simulink model "Chapter_4_Section_3_Model"  (R2017a)
settings: Solver=ode4  StartTime=0.0  StopTime=200  FixedStep=stp_sz  MaxStep=.0001  MinStep=.00005  RelTol=1e-7  AbsTol=1e-7  EnableMultiTasking=on
InitFcn:
  | load Chapter_4_Section_3
  | warning off
StopFcn:
  | save data.mat u_simulation v_simulation psi_simulation r_simulation npr_user_provided npr_achievable alpha_user_provided alpha_achievable stp_sz
  | clear all
  | load('data.mat')
  | delete('data.mat')
values from neighbouring files (symbols this model uses):
  A_disk = 13.2025431267    [Chapter_4_Section_3.mat]
  a_r11 = [-0.000865667853776 -0.901318756108 0.00874486630837 -0.00765974060328 0.00955717632387 0.00641813989061 -0.011076069832 0.00201248118094 -0.00501952733262 0.00315605586996 -0.00210851076531 0.0148609220099 ... (324 elements, 18x18)]    [Chapter_4_Section_3.mat]
  a_r13 = [-0.0294995912119 -4.91037219533 -0.00332739568397 0.0888755061346 -0.00681796875441 0.183812407485 0.0112008036726 0.10429312155 -0.0251601482875 -0.228675692165 0.00453476042855 0.0594697753606 ... (169 elements, 13x13)]    [Chapter_4_Section_3.mat]
  a_r15 = [-0.00127786555898 0.776225741104 -0.00474776997752 -0.00131066749835 0.0137520402687 -0.00211384579247 8.8019955143e-05 -0.00028996241197 -0.00129826872567 -0.0202543144732 0.0030370404199 -0.00453425604591 ... (169 elements, 13x13)]    [Chapter_4_Section_3.mat]
  a_r22 = [-0.000797108949019 -1.01015556887 0.00406573750109 -0.00111578544774 0.00423859757219 -0.00799128279013 0.00569024815652 -0.0167562674532 0.00334935655618 -0.000712432292804 0.00154242142086 0.00240437743229 ... (169 elements, 13x13)]    [Chapter_4_Section_3.mat]
  a_r24 = [-0.000686927823555 -0.95665602689 0.00244839898375 0.00145613314595 -0.00607023426216 0.0163996841317 0.00152022458075 -0.000736874734971 -0.00294919321651 -0.000761800577268 -0.00251686123035 -0.00197732815976 ... (169 elements, 13x13)]    [Chapter_4_Section_3.mat]
  a_r26 = [-0.194397873228 1.89810259721 -0.0873186628061 -0.241231729519 0.281206161775 -0.16994038615 -0.116565511469 -0.0496572593209 0.0216084469732 0.0912933167406 0.0299797727001 0.0314987707028 ... (169 elements, 13x13)]    [Chapter_4_Section_3.mat]
  a_r31 = [-0.00489112559449 -3.89960530455 -0.0361162658575 0.0265931197764 0.0034376033088 0.000316401308368 -0.0243996243526 0.0792200139858 -0.023187698537 -0.0726743997029 0.00400632061963 -0.0350516560041 ... (169 elements, 13x13)]    [Chapter_4_Section_3.mat]
  a_r33 = [-0.601431448276 0.50360246711 0.500115950342 -0.0452293844892 -0.0181314142185 -0.0323524621531 0.0355826051968 0.0329239610677 0.0940919952313 0.0566642992805 -0.0379178935102 0.0254835488846 ... (169 elements, 13x13)]    [Chapter_4_Section_3.mat]
  a_r35 = [-0.861988746714 -0.582511154549 0.34264856173 -0.0655310417272 -0.417167685168 0.183176698588 -0.473887691644 -0.225677727522 -0.133571139717 -0.218168843707 0.0850592077583 -0.0257492082836 ... (169 elements, 13x13)]    [Chapter_4_Section_3.mat]
  a_r42 = [-0.000411079312172 -0.966350953459 0.00419936729713 0.00358740198521 -0.00356571428733 -0.00958951498266 -0.00230062261745 -3.48708248632e-05 -0.00350313209064 -0.00772126326768 -0.0011918234528 -0.00149424537901 ... (169 elements, 13x13)]    [Chapter_4_Section_3.mat]
  a_r44 = [-0.000156115728087 -0.944139704333 -0.00242185567679 0.00620214191605 0.00232565005277 -0.00625050722164 0.00126021167241 -0.000681873506535 0.0011931592381 -0.00289361611357 -0.00138182415247 -0.00252837386868 ... (169 elements, 13x13)]    [Chapter_4_Section_3.mat]
  a_r46 = [-0.000218462457517 1.89677852742 0.00896242354968 -0.00290259500747 0.00225128874867 0.00254539590487 0.00120681433209 0.00261900930035 0.00149629742842 0.000796832004109 0.00199591847947 0.00352664402036 ... (169 elements, 13x13)]    [Chapter_4_Section_3.mat]
  a_r51 = [-0.0010898880101 0.776080724329 0.000225388678941 0.00375234840616 -0.00838297691459 -0.00447310416982 -0.0119510882322 -0.00692765468718 0.00227273345413 -0.0063592610709 0.000914007544175 0.00943534814934 ... (169 elements, 13x13)]    [Chapter_4_Section_3.mat]
  a_r53 = [-0.83377539904 0.569677058563 0.434285019976 0.157205409215 -0.397195569542 -0.255164078245 -0.141246880777 0.177451291189 -0.182828550566 0.0648162508754 0.244251292681 0.160100487197 ... (169 elements, 13x13)]    [Chapter_4_Section_3.mat]
  a_r55 = [-0.000352406331634 0.764343029796 0.00339830320259 -0.000678251137483 -0.00243783779313 -0.00215979913278 0.00196909451093 -0.00577428819561 -0.00349811892924 -0.00488920883323 0.00112064970343 0.000774855197444 ... (169 elements, 13x13)]    [Chapter_4_Section_3.mat]
  a_r62 = [-0.546519039316 -1.22303009993 0.393735845548 -0.120016588191 0.38151861373 -0.213578592342 -0.602267954372 -0.105716444149 -0.153151371839 -0.163939447448 -0.555540353196 0.0685401630267 ... (169 elements, 13x13)]    [Chapter_4_Section_3.mat]
  a_r64 = [-0.0406191100017 -5.18251105957 -0.115497941507 -0.0935821370219 0.180972853448 -0.0201998949456 -0.0698170640352 -0.0736823539521 -0.034828919888 0.0876659960431 -0.0419335596239 -0.0240984963396 ... (169 elements, 13x13)]    [Chapter_4_Section_3.mat]
  a_r66 = [-0.00276803466684 1.11530008029 0.0229779449181 0.0262185319857 0.00628472844795 0.000156167369042 -0.00250093023805 -0.0114435042874 -0.00826774415326 -0.00991601759993 -0.00812142854996 0.0148245002111 ... (169 elements, 13x13)]    [Chapter_4_Section_3.mat]
  A_rudder = 6    [Chapter_4_Section_3.mat]
  alpha_max = 0.392699081699    [Chapter_4_Section_3.mat]
  b_r11 = [-1.91804272115 -67.7547902158 12.3212653748 -6.25011871643 13.082442224 5.48501776184 -10.1596546398 2.56004852009 -4.74360113798 3.95981895348 -2.02856412397 18.3264246889 ... (18 elements, 18x1)]    [Chapter_4_Section_3.mat]
  b_r13 = [9.68113335046 8.54720242819 0.883931047444 -5.56576078332 1.72641800243 -13.8756826027 -2.702777864 -9.4621991361 5.92943514782 22.6516835054 -1.0074598861 -6.31102592982 ... (13 elements, 13x1)]    [Chapter_4_Section_3.mat]
  b_r22 = [-8.230214728 -263.156134326 24.2327808151 -4.87921448873 19.1715641288 -45.8768653263 26.6325387064 -91.9399975548 16.6663243552 -3.80929112747 7.68030110892 12.8381492859 ... (13 elements, 13x1)]    [Chapter_4_Section_3.mat]
  b_r24 = [20.6689502907 674.321335078 -41.3637763247 -19.2444203625 82.0775505272 -259.897803047 -22.2545830602 11.3827604156 43.2189922355 11.7516897475 36.9394390446 30.4503929007 ... (13 elements, 13x1)]    [Chapter_4_Section_3.mat]
  b_r26 = [206.794755218 -62.242559329 24.5666904254 184.158146246 -103.419961827 115.160111337 76.4499795128 20.3457431208 -13.1704465249 -41.5730935141 -18.1334448714 -14.4641153742 ... (13 elements, 13x1)]    [Chapter_4_Section_3.mat]
  b_r31 = [3.76230189948 5.16928151238 2.64945725635 -18.4251953385 -2.0625905672 -0.18887543415 4.20433084471 -14.07893046 13.0563354882 16.4007691754 -2.13849071942 8.28528512456 ... (13 elements, 13x1)]    [Chapter_4_Section_3.mat]
  b_r33 = [-425.265727934 16.4952177922 163.76327445 -15.539902078 -6.59006558263 -11.1862310226 12.8543123126 11.4260264426 33.8206936715 19.7626944669 -13.5783728882 8.91023495161 ... (13 elements, 13x1)]    [Chapter_4_Section_3.mat]
  b_r35 = [955.467057384 23.8174564739 -126.402446683 48.3788727465 168.435579445 -128.161344325 216.24493699 142.979450788 65.1193355403 134.911935543 -50.7648858119 13.1799100865 ... (13 elements, 13x1)]    [Chapter_4_Section_3.mat]
  b_r42 = [15.9360311823 665.959154186 -98.5777560157 -55.5400651809 61.9220987195 200.312325561 47.5124103398 0.631683490985 64.1219861023 155.750535985 22.3985447876 29.803792586 ... (13 elements, 13x1)]    [Chapter_4_Section_3.mat]
  b_r44 = [-27.1891200017 -1761.50772747 -283.391471232 367.311489951 182.522124626 -579.755911925 104.353356772 -62.2376848714 99.3185259533 -260.784153955 -116.536414334 -226.454300618 ... (13 elements, 13x1)]    [Chapter_4_Section_3.mat]
  b_r46 = [-26.6906838426 431.487773123 657.709356633 -144.976364483 114.646575538 180.775978583 85.0953284375 135.592940904 78.9082960716 55.2973047721 106.740201988 241.432567993 ... (13 elements, 13x1)]    [Chapter_4_Section_3.mat]
  b_r51 = [-27.9768378982 741.05041888 2.33758926296 57.3995096963 -127.005620965 -47.2947833409 -133.876425682 -98.5907202753 26.0445243962 -88.3721242204 10.7680008324 130.122749963 ... (13 elements, 13x1)]    [Chapter_4_Section_3.mat]
  b_r53 = [949.455593416 -23.2452293814 -157.318364745 -121.412853107 173.067821874 177.10214052 64.7164189373 -120.452255472 86.0623964314 -43.0643550932 -116.39314584 -105.497696438 ... (13 elements, 13x1)]    [Chapter_4_Section_3.mat]
  b_r55 = [-217.127382907 9506.32343029 1148.82922273 -188.742556573 -694.43970838 -709.996440288 566.872400877 -1877.38940059 -1026.37679575 -1566.80129668 332.089563592 247.692614281 ... (13 elements, 13x1)]    [Chapter_4_Section_3.mat]
  b_r62 = [259.61149635 16.5485296799 -38.0095496792 45.1883806678 -40.3107166739 78.3455844965 73.5107367495 37.0054960802 51.6709447748 22.7410486275 84.4875008959 -21.9559289205 ... (13 elements, 13x1)]    [Chapter_4_Section_3.mat]
  b_r64 = [156.539833252 187.686482031 376.820920142 59.4312894666 -548.902692032 17.0176436095 70.7484878223 206.821047291 37.1716677759 -243.032149857 114.824775027 27.0037475025 ... (13 elements, 13x1)]    [Chapter_4_Section_3.mat]
  b_r66 = [-314.266256408 5285.46587095 1093.01941502 1627.30071258 387.633965073 8.0986510694 -130.443621448 -701.343286032 -436.49966457 -600.0481003 -433.735518303 884.367320612 ... (13 elements, 13x1)]    [Chapter_4_Section_3.mat]
  bettas_CQ = [0 5.39 17.77 34.97 50.79 58.7 64.55 68.33 73.49 85.2 93.11 102.75 ... (40 elements, 1x40)]    [Chapter_4_Section_3.mat]    (also in looking_up_n.m = [0 5.39 17.77 34.97 50.79 58.7 64.55 68.33 73.49 85.2 93.11 )
  bettas_CT = [0 5.37 16.73 33.6 44.63 60.82 73.22 80.46 86.3 92.15 100.41 110.74 ... (52 elements, 1x52)]    [Chapter_4_Section_3.mat]    (also in looking_up_n.m = [0 5.37 16.73 33.6 44.63 60.82 73.22 80.46 86.3 92.15 100.41)
  c_r11 = [1.91804272142 -67.7547902158 -12.3212653748 -6.25011871643 -13.082442224 5.48501776185 -10.1596546398 -2.56004852009 -4.74360113798 -3.95981895348 -2.02856412396 -18.3264246889 ... (18 elements, 1x18)]    [Chapter_4_Section_3.mat]
  c_r13 = [9.68113335045 -8.54720242824 0.883931047418 5.56576078332 1.72641800244 13.8756826027 -2.702777864 9.4621991361 5.92943514781 -22.6516835054 -1.0074598861 6.31102592982 ... (13 elements, 1x13)]    [Chapter_4_Section_3.mat]
  c_r22 = [8.23021472807 -263.156134326 -24.2327808151 -4.87921448871 19.1715641288 45.8768653263 26.6325387064 91.9399975548 16.6663243552 3.80929112749 7.68030110892 -12.8381492859 ... (13 elements, 1x13)]    [Chapter_4_Section_3.mat]
  c_r24 = [20.6689502903 -674.321335078 -41.3637763247 19.2444203625 -82.0775505271 -259.897803047 22.2545830602 11.3827604156 -43.2189922355 11.7516897475 -36.9394390446 30.4503929007 ... (13 elements, 1x13)]    [Chapter_4_Section_3.mat]
  c_r26 = [-206.794755218 -62.2425593289 24.5666904254 -184.158146246 -103.419961827 -115.160111337 -76.4499795128 20.3457431209 13.1704465249 -41.5730935141 18.1334448714 -14.4641153742 ... (13 elements, 1x13)]    [Chapter_4_Section_3.mat]
  c_r31 = [3.76230189951 -5.16928151238 -2.64945725636 -18.4251953385 -2.0625905672 -0.188875434257 -4.2043308447 14.07893046 13.0563354882 -16.4007691754 -2.13849071943 -8.28528512456 ... (13 elements, 1x13)]    [Chapter_4_Section_3.mat]
  c_r33 = [-425.265727934 -16.4952177923 -163.76327445 15.539902078 -6.5900655826 11.1862310226 12.8543123126 -11.4260264426 33.8206936715 -19.7626944669 -13.5783728882 -8.91023495161 ... (13 elements, 1x13)]    [Chapter_4_Section_3.mat]
  c_r35 = [-955.467057384 23.8174564746 -126.402446683 -48.3788727464 168.435579445 128.161344325 216.24493699 -142.979450788 65.1193355403 -134.911935543 50.7648858119 13.1799100865 ... (13 elements, 1x13)]    [Chapter_4_Section_3.mat]
  c_r42 = [15.9360311824 -665.959154186 -98.5777560157 55.5400651809 -61.9220987195 200.312325561 47.5124103398 -0.631683490192 -64.1219861023 155.750535985 -22.3985447876 29.803792586 ... (13 elements, 1x13)]    [Chapter_4_Section_3.mat]
  c_r44 = [27.189120009 -1761.50772747 283.391471232 367.311489951 182.522124626 579.755911925 104.353356772 62.2376848713 99.3185259533 260.784153955 -116.536414334 226.454300618 ... (13 elements, 1x13)]    [Chapter_4_Section_3.mat]
  c_r46 = [26.6906838375 431.487773123 -657.709356633 -144.976364484 114.646575538 -180.775978583 -85.0953284373 135.592940904 78.9082960717 -55.297304772 106.740201988 -241.432567993 ... (13 elements, 1x13)]    [Chapter_4_Section_3.mat]
  c_r51 = [27.9768378982 741.05041888 2.33758926325 -57.3995096963 127.005620965 -47.2947833409 -133.876425682 98.5907202753 26.0445243962 88.3721242204 10.7680008324 -130.122749963 ... (13 elements, 1x13)]    [Chapter_4_Section_3.mat]
  c_r53 = [-949.455593416 -23.2452293814 -157.318364745 121.412853107 173.067821874 -177.10214052 64.7164189374 120.452255472 86.0623964314 43.0643550932 -116.39314584 105.497696438 ... (13 elements, 1x13)]    [Chapter_4_Section_3.mat]
  c_r55 = [217.12738291 9506.32343029 -1148.82922273 -188.742556576 -694.43970838 709.996440288 566.872400876 1877.38940059 -1026.37679575 1566.80129668 332.089563594 -247.69261428 ... (13 elements, 1x13)]    [Chapter_4_Section_3.mat]
  c_r62 = [-259.61149635 16.5485296799 -38.0095496792 -45.1883806678 -40.3107166739 -78.3455844965 73.5107367495 -37.0054960802 -51.6709447748 22.7410486275 84.4875008959 21.9559289205 ... (13 elements, 1x13)]    [Chapter_4_Section_3.mat]
  c_r64 = [-156.539833251 187.686482031 -376.820920142 59.4312894666 548.902692032 17.0176436097 70.7484878223 -206.82104729 37.1716677758 243.032149857 -114.824775027 27.0037475025 ... (13 elements, 1x13)]    [Chapter_4_Section_3.mat]
  c_r66 = [314.266256408 5285.46587095 1093.01941502 -1627.30071258 -387.633965073 8.09865107118 -130.443621448 701.343286032 -436.49966457 600.0481003 -433.735518303 -884.367320612 ... (13 elements, 1x13)]    [Chapter_4_Section_3.mat]
  CQs = [0.008 0.007 -0.002 -0.018 -0.037 -0.049 -0.06 -0.065 -0.068 -0.059 -0.057 -0.059 ... (40 elements, 1x40)]    [Chapter_4_Section_3.mat]    (also in looking_up_n.m = -0.1.*[-0.08 -0.07 0.02 0.18 0.37 0.49 0.6 0.65 0.68 0.59 0.)
  CTs = [0.32 0.29 0.19 0.01 -0.16 -0.46 -0.7 -0.77 -0.7 -0.63 -0.63 -0.69 ... (52 elements, 1x52)]    [Chapter_4_Section_3.mat]    (also in looking_up_n.m = [0.32 0.29 0.19 0.01 -0.16 -0.46 -0.7 -0.77 -0.7 -0.63 -0.63)
  d_r11 = 95.5285227708    [Chapter_4_Section_3.mat]
  d_r13 = -14.1628545989    [Chapter_4_Section_3.mat]
  d_r22 = 1468.51041279    [Chapter_4_Section_3.mat]
  d_r24 = -9785.77027698    [Chapter_4_Section_3.mat]
  d_r26 = -1700.92421833    [Chapter_4_Section_3.mat]
  d_r31 = -0.95522945761    [Chapter_4_Section_3.mat]
  d_r33 = 3827.81220596    [Chapter_4_Section_3.mat]
  d_r35 = -19539.5268707    [Chapter_4_Section_3.mat]
  d_r42 = -9418.04264727    [Chapter_4_Section_3.mat]
  d_r44 = 68252.1479072    [Chapter_4_Section_3.mat]
  d_r46 = -10162.1377852    [Chapter_4_Section_3.mat]
  d_r51 = 12054.4514237    [Chapter_4_Section_3.mat]
  d_r53 = -19539.5038011    [Chapter_4_Section_3.mat]
  d_r55 = 1991036.95813    [Chapter_4_Section_3.mat]
  d_r62 = -1405.47636444    [Chapter_4_Section_3.mat]
  d_r64 = -12342.2523681    [Chapter_4_Section_3.mat]
  d_r66 = 610786.440495    [Chapter_4_Section_3.mat]
  DEN = 5.34671106464e+28    [Chapter_4_Section_3.mat]
  dist_LOS = [-50 -49 -48 -47 -46 -45 -44 -43 -42 -41 -40 -39 ... (1051 elements, 1x1051)]    [Chapter_4_Section_3.mat]
  Dpr = 4.1    [Chapter_4_Section_3.mat]    (also in looking_up_n.m = u(4))
  Dw = 0.110526315789    [Chapter_4_Section_3.mat]
  dx = 10    [Chapter_4_Section_3.mat]
  dxr = 48.75    [Chapter_4_Section_3.mat]
  dy = 2    [Chapter_4_Section_3.mat]
  dz = 0.8    [Chapter_4_Section_3.mat]
  dzr = 0.514285714286    [Chapter_4_Section_3.mat]
  g = 10    [Chapter_4_Section_3.mat]
  gravity = 10    [Chapter_4_Section_3.mat]
  INDEX = [1 2 3 4 5 6 7 8 9]    [Chapter_4_Section_3.mat]
  Ix = 724554000    [Chapter_4_Section_3.mat]
  Iy = 4528460000    [Chapter_4_Section_3.mat]
  Iz = 4528460000    [Chapter_4_Section_3.mat]
  k_wave = [0.0157865285852 0.0224311321394 0.0345394916241 0.0578593033576 0.0778685019714 0.0983501894009 0.10403521245 0.134043066308 0.155236404606 0.203205074918 0.220032771713 0.262178651673 ... (20 elements, 1x20)]    [Chapter_4_Section_3.mat]
  Last_Pt_Accuracy = 30    [Chapter_4_Section_3.mat]
  LBP = 100    [Chapter_4_Section_3.mat]
  m = 7264000    [Chapter_4_Section_3.mat]
  phase = [4.61787442739 6.09845039199 5.44708367148 0.54182753101 2.30238916367 2.31974450279 4.30416083443 3.75697809799 4.95971993271 2.31003141527 1.29451121971 0.54454197722 ... (20 elements, 1x20)]    [Chapter_4_Section_3.mat]
  phi_0 = 0    [Chapter_4_Section_3.mat]
  psi_0 = 0    [Chapter_4_Section_3.mat]
  R_convrg = 220    [Chapter_4_Section_3.mat]
  radius_LOS = [166.575605377 166.637026665 166.698699321 166.760625342 166.82280675 166.885245588 166.947943925 167.010903854 167.074127493 167.137616985 167.201374499 167.265402228 ... (1051 elements, 1x1051)]    [Chapter_4_Section_3.mat]
  raw = 1000    [Chapter_4_Section_3.mat]    (also in looking_up_n.m = u(3))
  s = 0.15    [Chapter_4_Section_3.mat]
  S11 = 5.22457985714e+28    [Chapter_4_Section_3.mat]
  S13 = 3.79917831589e+26    [Chapter_4_Section_3.mat]
  S15 = -4.97006200608e+19    [Chapter_4_Section_3.mat]
  S22 = 4.58630932583e+28    [Chapter_4_Section_3.mat]
  S24 = 9.38800137353e+19    [Chapter_4_Section_3.mat]
  S26 = 1.30387886946e+18    [Chapter_4_Section_3.mat]
  S31 = 3.83422033136e+26    [Chapter_4_Section_3.mat]
  S33 = 1.77296018417e+28    [Chapter_4_Section_3.mat]
  S35 = 2.44593333777e+19    [Chapter_4_Section_3.mat]
  S42 = 8.93369784557e+19    [Chapter_4_Section_3.mat]
  S44 = 7.37931315974e+19    [Chapter_4_Section_3.mat]
  S46 = 27990784014.6    [Chapter_4_Section_3.mat]
  S51 = -4.98658939538e+19    [Chapter_4_Section_3.mat]
  S53 = 2.45188465874e+19    [Chapter_4_Section_3.mat]
  S55 = 1.18069051188e+19    [Chapter_4_Section_3.mat]
  S62 = 1.30580221388e+18    [Chapter_4_Section_3.mat]
  S64 = 23535167243.9    [Chapter_4_Section_3.mat]
  S66 = 1.18069078235e+19    [Chapter_4_Section_3.mat]
  ... (+18 more)
undefined symbols (not defined in the file or in its folder): magnitude
libraries: simulink x9
(part 3 of 6)

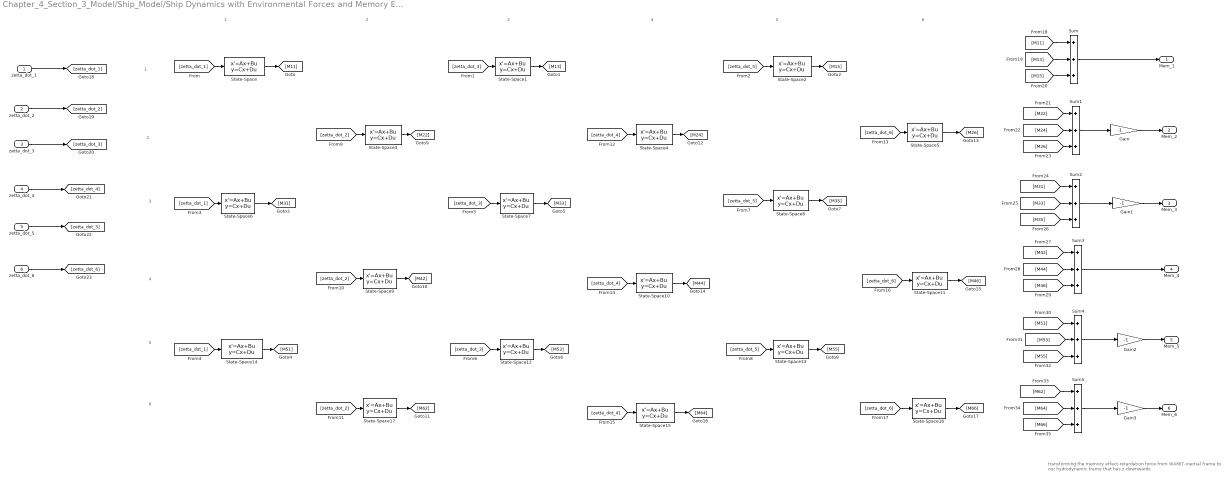
== system Chapter_4_Section_3_Model/Ship_Model/Ship Dynamics with Environmental Forces and Memory Effect/Memory effect using reduced order (13) state space representation(Kristiansen 2005)/Memory effect using reduced order (13) state space representation1 ==
  note: 1
  note: 2
  note: 3
  note: 4
  note: 5
  note: 6
  note: 1
  note: 2
  note: 3
  note: 4
  note: 5
  note: 6
  note: transforming the memory effect-retardation force from
      |  WAMIT-inertial frame to  our hydrodynamic
      |  frame that has z-downwards
  zetta_dot_1 : Inport
  zetta_dot_2 : Inport  Port=2
  zetta_dot_3 : Inport  Port=3
  zetta_dot_4 : Inport  Port=4
  zetta_dot_5 : Inport  Port=5
  zetta_dot_6 : Inport  Port=6
  Gain{,1..3} (4 alike) : Gain  Gain=-1
  State-Space : StateSpace  A=a_r11  B=b_r11  C=c_r11  D=d_r11  X0=0
  State-Space1 : StateSpace  A=a_r13  B=b_r13  C=c_r13  D=d_r13  X0=0
  State-Space10 : StateSpace  A=a_r44  B=b_r44  C=c_r44  D=d_r44  X0=0
  State-Space11 : StateSpace  A=a_r46  B=b_r46  C=c_r46  D=d_r46  X0=0
  State-Space12 : StateSpace  A=a_r53  B=b_r53  C=c_r53  D=d_r53  X0=0
  State-Space13 : StateSpace  A=a_r55  B=b_r55  C=c_r55  D=d_r55  X0=0
  State-Space14 : StateSpace  A=a_r51  B=b_r51  C=c_r51  D=d_r51  X0=0
  State-Space15 : StateSpace  A=a_r64  B=b_r64  C=c_r64  D=d_r64  X0=0
  State-Space16 : StateSpace  A=a_r66  B=b_r66  C=c_r66  D=d_r66  X0=0
  State-Space17 : StateSpace  A=a_r62  B=b_r62  C=c_r62  D=d_r62  X0=0
  State-Space2 : StateSpace  A=a_r15  B=b_r13  C=c_r13  D=d_r13  X0=0
  State-Space3 : StateSpace  A=a_r22  B=b_r22  C=c_r22  D=d_r22  X0=0
  State-Space4 : StateSpace  A=a_r24  B=b_r24  C=c_r24  D=d_r24  X0=0
  State-Space5 : StateSpace  A=a_r26  B=b_r26  C=c_r26  D=d_r26  X0=0
  State-Space6 : StateSpace  A=a_r31  B=b_r31  C=c_r31  D=d_r31  X0=0
  State-Space7 : StateSpace  A=a_r33  B=b_r33  C=c_r33  D=d_r33  X0=0
  State-Space8 : StateSpace  A=a_r35  B=b_r35  C=c_r35  D=d_r35  X0=0
  State-Space9 : StateSpace  A=a_r42  B=b_r42  C=c_r42  D=d_r42  X0=0
  Sum{,1..5} (6 alike) : Sum  Inputs=+++
  Mem_1 : Outport
  Mem_2 : Outport  Port=2
  Mem_3 : Outport  Port=3
  Mem_4 : Outport  Port=4
  Mem_5 : Outport  Port=5
  Mem_6 : Outport  Port=6
  wires:
  [zetta_dot_1] -> State-Space/1
  State-Space/1 -> [M11]
  [zetta_dot_3] -> State-Space1/1
  State-Space1/1 -> [M13]
  [zetta_dot_5] -> State-Space2/1
  State-Space2/1 -> [M15]
  [zetta_dot_1] -> State-Space6/1
  State-Space6/1 -> [M31]
  State-Space14/1 -> [M51]
  [zetta_dot_1] -> State-Space14/1
  [zetta_dot_3] -> State-Space7/1
  State-Space7/1 -> [M33]
  [zetta_dot_3] -> State-Space12/1
  State-Space12/1 -> [M53]
  [zetta_dot_5] -> State-Space8/1
  State-Space8/1 -> [M35]
  State-Space13/1 -> [M55]
  [zetta_dot_5] -> State-Space13/1
  [zetta_dot_2] -> State-Space3/1
  State-Space3/1 -> [M22]
  [zetta_dot_2] -> State-Space9/1
  State-Space9/1 -> [M42]
  [zetta_dot_2] -> State-Space17/1
  State-Space17/1 -> [M62]
  [zetta_dot_4] -> State-Space4/1
  [zetta_dot_4] -> State-Space10/1
  [zetta_dot_4] -> State-Space15/1
  [zetta_dot_6] -> State-Space5/1
  [zetta_dot_6] -> State-Space11/1
  [zetta_dot_6] -> State-Space16/1
  State-Space4/1 -> [M24]
  State-Space5/1 -> [M26]
  State-Space10/1 -> [M44]
  State-Space11/1 -> [M46]
  State-Space15/1 -> [M64]
  State-Space16/1 -> [M66]
  zetta_dot_1/1 -> [zetta_dot_1]
  zetta_dot_2/1 -> [zetta_dot_2]
  zetta_dot_3/1 -> [zetta_dot_3]
  zetta_dot_4/1 -> [zetta_dot_4]
  zetta_dot_5/1 -> [zetta_dot_5]
  zetta_dot_6/1 -> [zetta_dot_6]
  [M11] -> Sum/1
  [M13] -> Sum/2
  [M15] -> Sum/3
  Sum/1 -> Mem_1/1
  [M22] -> Sum1/1
  [M24] -> Sum1/2
  [M26] -> Sum1/3
  Sum1/1 -> Gain/1
  [M31] -> Sum2/1
  [M33] -> Sum2/2
  [M35] -> Sum2/3
  Sum2/1 -> Gain1/1
  Sum3/1 -> Mem_4/1
  [M42] -> Sum3/1
  [M44] -> Sum3/2
  [M46] -> Sum3/3
  [M51] -> Sum4/1
  [M53] -> Sum4/2
  [M55] -> Sum4/3
  Sum4/1 -> Gain2/1
  [M62] -> Sum5/1
  [M64] -> Sum5/2
  [M66] -> Sum5/3
  Sum5/1 -> Gain3/1
  Gain/1 -> Mem_2/1
  Gain1/1 -> Mem_3/1
  Gain2/1 -> Mem_5/1
  Gain3/1 -> Mem_6/1

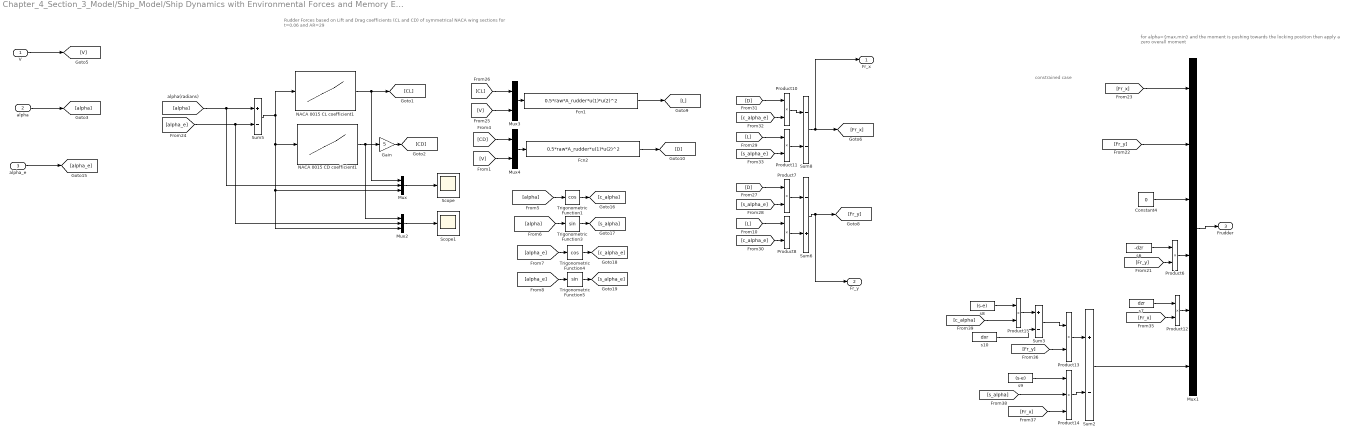
== system Chapter_4_Section_3_Model/Ship_Model/Ship Dynamics with Environmental Forces and Memory Effect/Rudder/Rudder Dynamics ==
  note: Rudder Forces based on  Lift and Drag coefficients (CL and CD)
      | of symmetrical NACA wing sections for t=0.06 and AR=29
  note: constrained case
  note: for alpha={max,min} and the moment is pushing towards
      |  the locking position then apply a zero overall moment
  V : Inport
  alpha : Inport  Port=2
  alpha_e : Inport  Port=3
  Constant4 : Constant  Value=0
  Fcn1 : Fcn  Expr=0.5*raw*A_rudder*u(1)*u(2)^2
  Fcn2 : Fcn  Expr=0.5*raw*A_rudder*u(1)*u(2)^2
  Gain : Gain  Gain=5
  Mux : Mux  Inputs=3
  Mux1 : Mux  Inputs=6
  Mux2 : Mux  Inputs=3
  Mux3 : Mux  Inputs=2
  Mux4 : Mux  Inputs=2
  NACA 0015 CD coefficient1 : Lookup  InputValues="[-0.5236   -0.4189   -0.3491   -0.2793   -0.2094   -0.1396   -0.0698         0   0.0698    0.1396    0.2094    0.2793    0.3491    0.4189    0.5236]"  Table="[0.5140    0.2400    0.1410    0.0980    0.0600    0.0360    0.0180    0.0150  0.0180    0.0360    0.0600    0.0980    0.1410    0.2400    0.5140]"  LookUpMeth=Interpolation-Use End Values  RndMeth=Nearest
  NACA 0015 CL coefficient1 : Lookup  InputValues="[-3.926990816987241e-001   -3.490658503988659e-001   -2.792526803190927e-001   -2.094395102393195e-001   -1.396263401595464e-001   -6.981317007977318e-002   0   6.981317007977318e-002    1.396263401595464e-001    2.094395102393195e-001    2.792526803190927e-001    3.490658503988659e-001    3.926990816987241e-001]"  Table="[-1.500000000000000e+000   -1.420000000000000e+000   -1.140000000000000e+000   -8.900000000000000e-001   -6.100000000000000e-001   -3.000000000000000e-001 0   3.000000000000000e-001    6.100000000000000e-001    8.900000000000000e-001    1.140000000000000e+000    1.420000000000000e+000    1.500000000000000e+000]"  LookUpMeth=Interpolation-Use End Values  RndMeth=Nearest
  Product{6..8,10..13,15} (8 alike) : Product  RndMeth=Zero
  Product14 : Product  Inputs=3  RndMeth=Zero
  Scope : Scope
  Scope1 : Scope
  Sum2 : Sum  Inputs=+-
  Sum3 : Sum  Inputs=+-
  Sum5 : Sum  Inputs=+-
  Sum6 : Sum  Inputs=-+
  Sum8 : Sum  Inputs=--
  Trigonometric Function1 : Trigonometry  Operator=cos
  Trigonometric Function3 : Trigonometry
  Trigonometric Function4 : Trigonometry  Operator=cos
  Trigonometric Function5 : Trigonometry
  s10 : Constant  Value=dxr
  s6 : Constant  Value=-dzr
  s7 : Constant  Value=dzr
  s8 : Constant  Value=(s-e)
  s9 : Constant  Value=(s-e)
  Fr_x : Outport
  Fr_y : Outport  Port=2
  Frudder : Outport  Port=3
  wires:
  Fcn1/1 -> [L]
  V/1 -> [V]
  NACA 0015 CL coefficient1/1 -> Mux/1, [CL]
  NACA 0015 CD coefficient1/1 -> Mux2/1, Gain/1
  [alpha_e] -> Mux2/2, Sum5/2
  [CL] -> Mux3/1
  [V] -> Mux3/2
  Mux3/1 -> Fcn1/1
  [CD] -> Mux4/1
  [V] -> Mux4/2
  Mux4/1 -> Fcn2/1
  Fcn2/1 -> [D]
  [alpha] -> Trigonometric Function1/1
  Trigonometric Function1/1 -> [c_alpha]
  [alpha] -> Trigonometric Function3/1
  Trigonometric Function3/1 -> [s_alpha]
  [alpha_e] -> Trigonometric Function4/1
  Trigonometric Function4/1 -> [c_alpha_e]
  [alpha_e] -> Trigonometric Function5/1
  Trigonometric Function5/1 -> [s_alpha_e]
  [D] -> Product7/1
  [s_alpha_e] -> Product7/2
  Product7/1 -> Sum6/1
  [L] -> Product8/1
  [c_alpha_e] -> Product8/2
  Product8/1 -> Sum6/2
  [D] -> Product10/1
  [c_alpha_e] -> Product10/2
  Product10/1 -> Sum8/1
  [L] -> Product11/1
  [s_alpha_e] -> Product11/2
  Product11/1 -> Sum8/2
  Sum8/1 -> [Fr_x], Fr_x/1
  Sum6/1 -> [Fr_y], Fr_y/1
  s6/1 -> Product6/1
  [Fr_y] -> Product6/2
  [Fr_x] -> Mux1/1
  [Fr_y] -> Mux1/2
  s7/1 -> Product12/1
  [Fr_x] -> Product12/2
  Constant4/1 -> Mux1/3
  Product6/1 -> Mux1/4
  Product12/1 -> Mux1/5
  Mux1/1 -> Frudder/1
  Product13/1 -> Sum2/1
  s9/1 -> Product14/1
  [s_alpha] -> Product14/2
  [Fr_x] -> Product14/3
  s8/1 -> Product15/1
  [c_alpha] -> Product15/2
  Product15/1 -> Sum3/1
  s10/1 -> Sum3/2
  Sum3/1 -> Product13/1
  [Fr_y] -> Product13/2
  Product14/1 -> Sum2/2
  Sum2/1 -> Mux1/6
  [alpha] -> Mux/2, Sum5/1
  alpha/1 -> [alpha]
  alpha_e/1 -> [alpha_e]
  Sum5/1 -> Mux2/3, Mux/3, NACA 0015 CD coefficient1/1, NACA 0015 CL coefficient1/1
  Mux/1 -> Scope/1
  Mux2/1 -> Scope1/1
  Gain/1 -> [CD]

== system Chapter_4_Section_3_Model/Ship_Model/Ship Dynamics with Environmental Forces and Memory Effect/Six DOF State Integrator of the Ship/Subsystem ==
  In1 : Inport
  Constant10 : Constant  Value=Iy
  Constant11 : Constant  Value=Iz
  Constant{6..8,12,14} (5 alike) : Constant  Value=0
  Constant13 : Constant  Value=DEN
  Constant15 : Constant  Value=m
  Constant31 : Constant  Value=S26
  Constant32 : Constant  Value=S35
  Constant35 : Constant  Value=S33
  Constant36 : Constant  Value=S31
  Constant39 : Constant  Value=S46
  Constant40 : Constant  Value=S13
  Constant41 : Constant  Value=S42
  Constant44 : Constant  Value=S44
  Constant47 : Constant  Value=S66
  Constant48 : Constant  Value=S11
  Constant50 : Constant  Value=S53
  Constant51 : Constant  Value=S15
  Constant52 : Constant  Value=S51
  Constant54 : Constant  Value=S55
  Constant56 : Constant  Value=S62
  Constant59 : Constant  Value=S64
  Constant61 : Constant  Value=S22
  Constant64 : Constant  Value=S24
  Constant9 : Constant  Value=Ix
  Demux4 : Demux  Outputs=6
  Mux1 : Mux  Inputs=35
  S-Function Builder : S-Function  FunctionName=state_space_c  SFunctionModules=state_space_c_wrapper  SFunctionDeploymentMode=off  EnableBusSupport=off  mask(S-Function Builder){}
      mask init:
      | val = [[.9  0.75 0.75 1 1 .9 .9 1]',[1 1 0.75 0.75 .9 .9 1 .9]'];try , sys = get_param(gcb,'SfunBuilderFcnName');if isempty(sys), sys = get_param(gcb,'FunctionName'); end,catch, sys = get_param(gcb,'FunctionName'); end
      settings: CopyFcn=set_param(gcbh,'LinkStatus','none')  PreSaveFcn=try, set_param(gcb,'FunctionName','state_space_c'), end  OpenFcn=sfunctionwizard(gcbh)
      mask Display: plot(val(:,1),val(:,2)),disp(sys), port_label('input',1,'u0'), port_label('output',1,'y0')
  Out1 : Outport
  wires:
  Demux4/1 -> Mux1/1
  Demux4/2 -> Mux1/2
  Demux4/6 -> Mux1/6
  Constant7/1 -> Mux1/7
  Constant6/1 -> Mux1/8
  Constant8/1 -> Mux1/9
  Constant9/1 -> Mux1/10
  Constant10/1 -> Mux1/11
  Constant11/1 -> Mux1/12
  Constant12/1 -> Mux1/13, Mux1/14
  Constant14/1 -> Mux1/15
  Constant15/1 -> Mux1/16
  Demux4/3 -> Mux1/3
  Demux4/4 -> Mux1/4
  Demux4/5 -> Mux1/5
  Constant48/1 -> Mux1/17
  Constant40/1 -> Mux1/18
  Constant51/1 -> Mux1/19
  Constant61/1 -> Mux1/20
  Constant64/1 -> Mux1/21
  Constant31/1 -> Mux1/22
  Constant36/1 -> Mux1/23
  Constant35/1 -> Mux1/24
  Constant32/1 -> Mux1/25
  Constant41/1 -> Mux1/26
  Constant44/1 -> Mux1/27
  Constant39/1 -> Mux1/28
  Constant52/1 -> Mux1/29
  Constant50/1 -> Mux1/30
  Constant54/1 -> Mux1/31
  Constant56/1 -> Mux1/32
  Constant59/1 -> Mux1/33
  Constant47/1 -> Mux1/34
  Constant13/1 -> Mux1/35
  In1/1 -> Demux4/1
  S-Function Builder/1 -> Out1/1
  Mux1/1 -> S-Function Builder/1

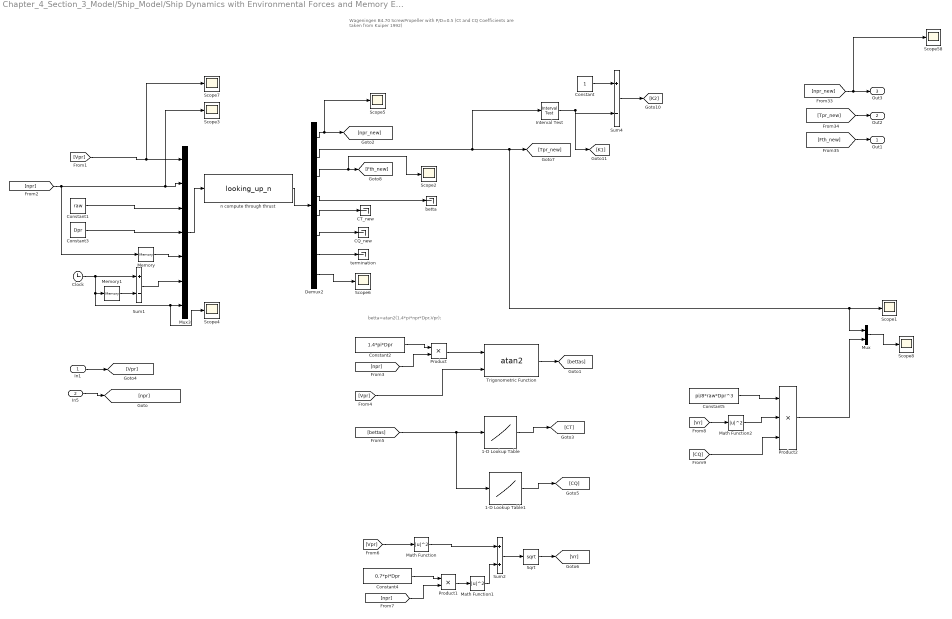
== system Chapter_4_Section_3_Model/Ship_Model/Ship Dynamics with Environmental Forces and Memory Effect/Subsystem3/Subsystem ==
  note: betta=atan2(1.4*pi*npr*Dpr,Vpr);
  note: Wageningen B4.70 ScrewPropeller with P/D=0.5
      |  (Ct and CQ Coefficients are taken from Kuiper 1992)
  In1 : Inport
  In5 : Inport  Port=2
  1-D Lookup Table : Lookup_n-D  NumberOfTableDimensions=1  BreakpointsForDimension1=bettas_CT  Table=CTs  ExtrapMethod=Clip  InternalRulePriority=Speed  RndMeth=Simplest  InputSameDT=on
  1-D Lookup Table1 : Lookup_n-D  NumberOfTableDimensions=1  BreakpointsForDimension1=bettas_CQ  Table=CQs  ExtrapMethod=Clip  InternalRulePriority=Speed  RndMeth=Simplest  InputSameDT=on
  CQ_new : Terminator
  CT_new : Terminator
  Clock : Clock
  Constant : Constant
  Constant1 : Constant  Value=raw
  Constant2 : Constant  Value=1.4*pi*Dpr
  Constant3 : Constant  Value=Dpr
  Constant4 : Constant  Value=0.7*pi*Dpr
  Constant5 : Constant  Value=pi/8*raw*Dpr^3
  Demux2 : Demux  Outputs=8
  Interval Test : simulink/Logic and Bit Operations/Interval Test  IntervalClosedRight=on  uplimit=Tmax  IntervalClosedLeft=on  lowlimit=Tmin  OutDataTypeStr=uint8
  Math Function : Math  Operator=magnitude^2  SaturateOnIntegerOverflow=on
  Math Function1 : Math  Operator=magnitude^2  SaturateOnIntegerOverflow=on
  Math Function2 : Math  Operator=magnitude^2  SaturateOnIntegerOverflow=on
  Memory : Memory  X0=10
  Memory1 : Memory  X0=-0.01
  Mux : Mux  Inputs=2
  Mux3 : Mux  Inputs=7
  Product : Product
  Product1 : Product
  Product2 : Product  Inputs=3
  Scope{1..8,58} (9 alike) : Scope
  Sqrt : Sqrt  SaturateOnIntegerOverflow=on
  Sum1 : Sum  Inputs=+-
  Sum2 : Sum
  Sum4 : Sum  Inputs=|+|-|
  Trigonometric Function : Trigonometry  Operator=atan2
  betta : Terminator
  n compute through thrust : S-Function  FunctionName=looking_up_n  SFunctionDeploymentMode=off  EnableBusSupport=off
  termination : Terminator
  Out1 : Outport
  Out2 : Outport  Port=2
  Out3 : Outport  Port=3
  wires:
  In5/1 -> [npr]
  In1/1 -> [Vpr]
  Interval Test/1 -> Sum4/2, [K1]
  Sum4/1 -> [K2]
  [npr_new] -> Scope58/1, Out3/1
  [Tpr_new] -> Out2/1
  [Fth_new] -> Out1/1
  Constant/1 -> Sum4/1
  Demux2/6 -> CQ_new/1
  Constant1/1 -> Mux3/3
  Constant3/1 -> Mux3/4
  [Vpr] -> Scope7/1, Mux3/1
  Mux3/1 -> n compute through thrust/1
  n compute through thrust/1 -> Demux2/1
  Demux2/1 -> [npr_new], Scope5/1
  Demux2/2 -> Interval Test/1, [Tpr_new], Mux/1, Scope1/1
  Demux2/3 -> Scope2/1, [Fth_new]
  Demux2/4 -> betta/1
  Demux2/5 -> CT_new/1
  Demux2/7 -> termination/1
  [npr] -> Memory/1, Scope3/1, Mux3/2
  Clock/1 -> Scope4/1, Mux3/7, Memory1/1, Sum1/1
  Memory1/1 -> Sum1/2
  Memory/1 -> Mux3/5
  Sum1/1 -> Mux3/6
  Demux2/8 -> Scope6/1
  Constant2/1 -> Product/1
  [npr] -> Product/2
  Product/1 -> Trigonometric Function/1
  [Vpr] -> Trigonometric Function/2
  Trigonometric Function/1 -> [bettas]
  [bettas] -> 1-D Lookup Table1/1, 1-D Lookup Table/1
  1-D Lookup Table/1 -> [CT]
  1-D Lookup Table1/1 -> [CQ]
  [Vpr] -> Math Function/1
  Math Function/1 -> Sum2/1
  [npr] -> Product1/2
  Constant4/1 -> Product1/1
  Product1/1 -> Math Function1/1
  Math Function1/1 -> Sum2/2
  Sum2/1 -> Sqrt/1
  Sqrt/1 -> [Vr]
  Constant5/1 -> Product2/1
  [Vr] -> Math Function2/1
  Math Function2/1 -> Product2/2
  Product2/1 -> Mux/2
  Mux/1 -> Scope8/1
  [CQ] -> Product2/3

== system Chapter_4_Section_3_Model/Ship_Model/Ship Dynamics with Environmental Forces and Memory Effect/Wave Excitation Force/wave elevation from multiple frequencies2 ==
  X : Inport
  Y : Inport  Port=2
  angle : Inport  Port=3
  ksi : Inport  Port=4
  Clock : Clock
  Constant2 : Constant
  Gain4 : Gain  Gain=0.1
  Gain5 : Gain  Gain=10
  Rounding Function3 : Rounding  Operator=round
  "Seakeeping motion of the ship from RAO's and wave spectrum " : Subsystem  TreatAsAtomicUnit=on
  F : Outport
  wires:
  Constant2/1 -> "Seakeeping motion of the ship from RAO's and wave spectrum "/1(IC)
  Clock/1 -> "Seakeeping motion of the ship from RAO's and wave spectrum "/4(t)
  X/1 -> "Seakeeping motion of the ship from RAO's and wave spectrum "/2(X)
  "Seakeeping motion of the ship from RAO's and wave spectrum "/1(F) -> F/1
  Y/1 -> "Seakeeping motion of the ship from RAO's and wave spectrum "/3(Y)
  Gain4/1 -> Rounding Function3/1
  Rounding Function3/1 -> Gain5/1
  angle/1 -> Gain4/1
  Gain5/1 -> "Seakeeping motion of the ship from RAO's and wave spectrum "/5(angle)
  ksi/1 -> "Seakeeping motion of the ship from RAO's and wave spectrum "/6(ksi)

== system Chapter_4_Section_3_Model/Ship_Model/Ship Dynamics with Environmental Forces and Memory Effect/Wind Force/wind force ==
  note: This block computes the wind coefficients using the method of Isherwood.
      | Inputs: wind angle(degrees)(0-360)
      |             ship type: integer 1-11
      | Outputs: [Cx ;Cy; Cxy]
  note: deg
  relative wind angle_degree : Inport
  relative velocity of the wind (m/s) : Inport  Port=2
  Embedded MATLAB Function2 : MATLAB Function  Description="This function computes the three wind coefficients based on Isherwood's  method (1973) for ships with unknown dimension paramters."  TreatAsAtomicUnit=on
  Subsystem : Subsystem
  ship type : Constant  Value=11
  ship type11 : Constant  Value=100
  ship type12 : Constant  Value=320
  ship type13 : Constant  Value=64
  ship type9 : Constant  Value=1.28
  F_wind : Outport
  wires:
  ship type/1 -> Embedded MATLAB Function2/2(Ship_type)
  ship type9/1 -> Subsystem/4(density of air)
  ship type11/1 -> Subsystem/6("LOA: overall length ")
  ship type12/1 -> Subsystem/8(AL: lateral projected area)
  ship type13/1 -> Subsystem/7(AT: transverse projected area1)
  relative wind angle_degree/1 -> Embedded MATLAB Function2/1(Wind_angle)
  Subsystem/1(F_wind) -> F_wind/1
  relative velocity of the wind (m/s)/1 -> Subsystem/5(velocity of the wind)
  Embedded MATLAB Function2/1(Cxw) -> Subsystem/1(Cx)
  Embedded MATLAB Function2/2(Cyw) -> Subsystem/2(Cy)
  Embedded MATLAB Function2/3(CNw) -> Subsystem/3(Cxy)

== system Chapter_4_Section_3_Model/Ship_Model/Ship Dynamics with Environmental Forces and Memory Effect/Buoyancy_Forces/Subsystem/If Action Subsystem ==
  Action Port : ActionPort  PropagateVarSize=During execution  ActionType=then
  Constant : Constant  Value=0
  Constant1 : Constant  Value=0
  Constant2 : Constant  Value=0
  Out1 : Outport
  Out2 : Outport  Port=2
  Out3 : Outport  Port=3
  wires:
  Constant/1 -> Out1/1
  Constant1/1 -> Out2/1
  Constant2/1 -> Out3/1

== system Chapter_4_Section_3_Model/Ship_Model/Ship Dynamics with Environmental Forces and Memory Effect/Buoyancy_Forces/Subsystem/If Action Subsystem1 ==
  xb : Inport
  yb : Inport  Port=2
  zb : Inport  Port=3
  Vsub : Inport  Port=4
  Action Port : ActionPort  PropagateVarSize=During execution  ActionType=else
  Product1 : Product  Inputs=/*  RndMeth=Zero
  Product2 : Product  Inputs=/*  RndMeth=Zero
  Product3 : Product  Inputs=/*  RndMeth=Zero
  Out1 : Outport
  Out2 : Outport  Port=2
  Out3 : Outport  Port=3
  wires:
  xb/1 -> Product1/2
  yb/1 -> Product2/2
  zb/1 -> Product3/2
  Vsub/1 -> Product1/1, Product2/1, Product3/1
  Product1/1 -> Out1/1
  Product2/1 -> Out2/1
  Product3/1 -> Out3/1

== system Chapter_4_Section_3_Model/Ship_Model/Ship Dynamics with Environmental Forces and Memory Effect/Buoyancy_Forces/Subsystem/wave elevation from multiple frequencies ==
  X : Inport
  Y : Inport  Port=2
  ksi : Inport  Port=3
  Clock : Clock
  Constant2 : Constant
  "Seakeeping motion of the ship from RAO's and wave spectrum " : Subsystem  TreatAsAtomicUnit=on
  taw : Outport
  wires:
  Constant2/1 -> "Seakeeping motion of the ship from RAO's and wave spectrum "/1(IC)
  Clock/1 -> "Seakeeping motion of the ship from RAO's and wave spectrum "/4(t)
  X/1 -> "Seakeeping motion of the ship from RAO's and wave spectrum "/2(X)
  "Seakeeping motion of the ship from RAO's and wave spectrum "/1(taw) -> taw/1
  Y/1 -> "Seakeeping motion of the ship from RAO's and wave spectrum "/3(Y)
  ksi/1 -> "Seakeeping motion of the ship from RAO's and wave spectrum "/5(ksi)

== system Chapter_4_Section_3_Model/Ship_Model/Ship Dynamics with Environmental Forces and Memory Effect/Buoyancy_Forces/Subsystem/wave elevation from multiple frequencies1 ==
  X : Inport
  Y : Inport  Port=2
  ksi : Inport  Port=3
  Clock : Clock
  Constant2 : Constant
  "Seakeeping motion of the ship from RAO's and wave spectrum " : Subsystem  TreatAsAtomicUnit=on
  taw : Outport
  wires:
  Constant2/1 -> "Seakeeping motion of the ship from RAO's and wave spectrum "/1(IC)
  Clock/1 -> "Seakeeping motion of the ship from RAO's and wave spectrum "/4(t)
  X/1 -> "Seakeeping motion of the ship from RAO's and wave spectrum "/2(X)
  "Seakeeping motion of the ship from RAO's and wave spectrum "/1(taw) -> taw/1
  Y/1 -> "Seakeeping motion of the ship from RAO's and wave spectrum "/3(Y)
  ksi/1 -> "Seakeeping motion of the ship from RAO's and wave spectrum "/5(ksi)

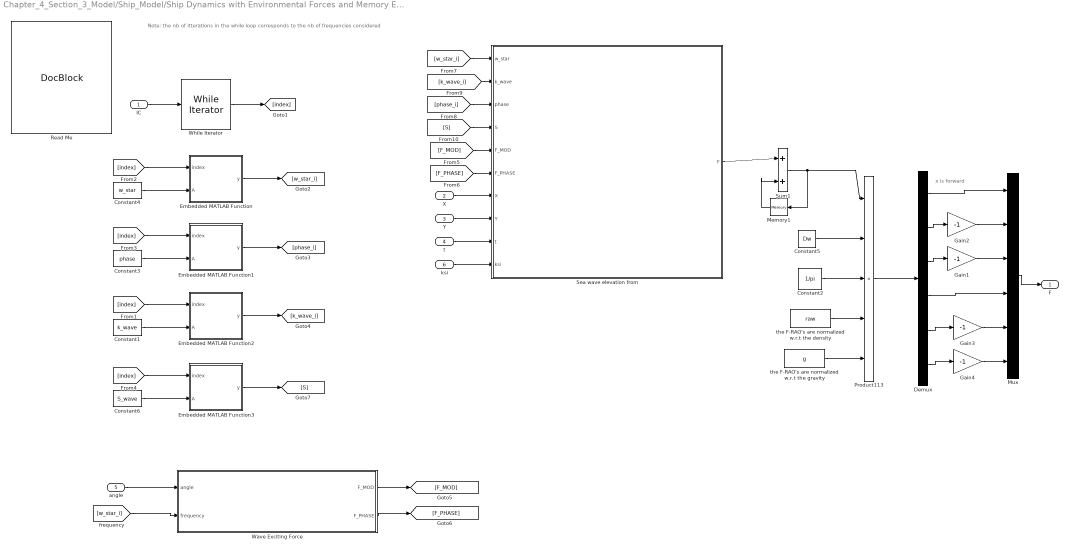
== system Chapter_4_Section_3_Model/Ship_Model/Ship Dynamics with Environmental Forces and Memory Effect/Wave Excitation Force/wave elevation from multiple frequencies2/Seakeeping motion of the ship from RAO's and wave spectrum  ==
  note: Note: the nb of itterations in the while loop corresponds to the nb of frequencies considered
  note: x is forward
  IC : Inport
  X : Inport  Port=2
  Y : Inport  Port=3
  t : Inport  Port=4
  angle : Inport  Port=5
  ksi : Inport  Port=6
  Constant1 : Constant  Value=k_wave
  Constant2 : Constant  Value=1/pi
  Constant3 : Constant  Value=phase
  Constant4 : Constant  Value=w_star
  Constant5 : Constant  Value=Dw
  Constant6 : Constant  Value=S_wave
  Demux : Demux  Outputs=6
  Embedded MATLAB Function : MATLAB Function  TreatAsAtomicUnit=on
  Embedded MATLAB Function1 : MATLAB Function  TreatAsAtomicUnit=on
  Embedded MATLAB Function2 : MATLAB Function  TreatAsAtomicUnit=on
  Embedded MATLAB Function3 : MATLAB Function  TreatAsAtomicUnit=on
  Gain{1..4} (4 alike) : Gain  Gain=-1
  Memory1 : Memory  X0=[0 0 0 0 0 0]  InheritSampleTime=on
  Mux : Mux  Inputs=6
  Product113 : Product  Inputs=5  RndMeth=Zero
  Read Me : simulink/Model-Wide Utilities/DocBlock  DocumentType=Text
      content=|
      | This subsystem computes the surge, sway, heave, roll, pitch and yaw motions of the center of the body fixed frame.
      | The elevation of the sea wave is given by the ITTC_Modified_Pierson_Moskowitz spectrum.
      | Inputs are:
      | w_star: frequency of the wave (chosen randomly between [wn-Dw/2,wn+Dw/2] offline prior to simulation)
      | phase: phase angle of the wave(chosen randomly between [0,2pi] offline prior to simulation)
      | ksi: direction of the wave(one angle for long crested sea, offline prior to simulation)
      | U: speed of the ship [m/s]-varying with time
      | psi: yaw angle of the ship==heading[rad] -varying with time
      | time: seconds
      | k_wave_i:wave number(computed offline before the simulation)
      | x:surge location of the ship w.r.t the inertial frame
      | y:sway location of the ship w.r.t the inertial frame
      |
      | WAMIT inertial frame is different than our hydrodynamic frame(z is upwards in WAMIT)
      |
      |
      |
      | WAMIT inertial frame:
      |                z
      |                *            y
      |                *           *
      |                *        *
      |                *      *
      |                *   *
      |                *   *   *   *   *   *   *   *   * x
      |
      |
      | after computing the surge, sway, heave, roll, pitch and yaw motions of the center of the body fixed frame, one has to transform those
      | quantities to the hydrodynamic frame(z-downward)
      | surge==surge
      | sway== - sway
      | heave== - heave
      | roll==roll
      | pitch=-pitch
      | yaw=-yaw
  "Sea wave elevation from " : Subsystem
  Sum1 : Sum  Inputs=|+|+|
  Wave Exciting Force : Subsystem
  While Iterator : WhileIterator  MaxIters=20  WhileBlockType=do-while  ResetStates=reset  ShowIterationPort=on  OutputDataType=double
  the F-RAO's are normalized w.r.t the density : Constant  Value=raw
  the F-RAO's are normalized w.r.t the gravity : Constant  Value=g
  F : Outport
  wires:
  While Iterator/1 -> [index]
  IC/1 -> While Iterator/1
  [index] -> Embedded MATLAB Function/1(index)
  Constant4/1 -> Embedded MATLAB Function/2(A)
  Embedded MATLAB Function/1(y) -> [w_star_i]
  [index] -> Embedded MATLAB Function1/1(index)
  Constant3/1 -> Embedded MATLAB Function1/2(A)
  Embedded MATLAB Function1/1(y) -> [phase_i]
  [index] -> Embedded MATLAB Function2/1(index)
  Constant1/1 -> Embedded MATLAB Function2/2(A)
  Embedded MATLAB Function2/1(y) -> [k_wave_i]
  [w_star_i] -> "Sea wave elevation from "/1(w_star)
  [k_wave_i] -> "Sea wave elevation from "/2(k_wave)
  [phase_i] -> "Sea wave elevation from "/3(phase)
  X/1 -> "Sea wave elevation from "/7(X)
  Y/1 -> "Sea wave elevation from "/8(Y)
  "Sea wave elevation from "/1(F) -> Sum1/1
  Sum1/1 -> Memory1/1, Product113/1
  Memory1/1 -> Sum1/2
  t/1 -> "Sea wave elevation from "/9(t)
  [w_star_i] -> Wave Exciting Force/2(frequency)
  angle/1 -> Wave Exciting Force/1(angle)
  Wave Exciting Force/1("F_MOD ") -> [F_MOD]
  Wave Exciting Force/2("F_PHASE ") -> [F_PHASE]
  Constant2/1 -> Product113/3
  the F-RAO's are normalized w.r.t the density/1 -> Product113/4
  the F-RAO's are normalized w.r.t the gravity/1 -> Product113/5
  Constant5/1 -> Product113/2
  [F_MOD] -> "Sea wave elevation from "/5(F_MOD)
  [F_PHASE] -> "Sea wave elevation from "/6("F_PHASE ")
  Product113/1 -> Demux/1
  Mux/1 -> F/1
  Demux/1 -> Mux/1
  Demux/2 -> Gain2/1
  Gain2/1 -> Mux/2
  Demux/3 -> Gain1/1
  Gain1/1 -> Mux/3
  Demux/4 -> Mux/4
  Demux/5 -> Gain3/1
  Gain3/1 -> Mux/5
  Demux/6 -> Gain4/1
  Gain4/1 -> Mux/6
  [index] -> Embedded MATLAB Function3/1(index)
  Constant6/1 -> Embedded MATLAB Function3/2(A)
  Embedded MATLAB Function3/1(y) -> [S]
  [S] -> "Sea wave elevation from "/4(S)
  ksi/1 -> "Sea wave elevation from "/10(ksi)

== system Chapter_4_Section_3_Model/Ship_Model/Ship Dynamics with Environmental Forces and Memory Effect/Wind Force/wind force/Subsystem ==
  Cx : Inport
  Cy : Inport  Port=2
  Cxy : Inport  Port=3
  density of air : Inport  Port=4
  velocity of the wind : Inport  Port=5
  "LOA: overall length " : Inport  Port=6
  AT: transverse projected area1 : Inport  Port=7
  AL: lateral projected area : Inport  Port=8
  Constant : Constant  Value=0.5
  Constant1 : Constant  Value=0.5
  Constant3 : Constant  Value=0.5
  Constant4 : Constant  Value=0
  Constant5 : Constant  Value=0
  Constant6 : Constant  Value=0
  Mux1 : Mux  Inputs=6
  Product : Product  Inputs=6  RndMeth=Zero
  Product1 : Product  Inputs=6  RndMeth=Zero
  Product3 : Product  Inputs=7  RndMeth=Zero
  transform z-downwards : Gain  Gain=-1
  F_wind : Outport
  wires:
  Constant/1 -> Product/1
  [Cx] -> Product/2
  [r_air] -> Product/3
  [Vw] -> Product/4
  [Vw] -> Product/5
  [AT] -> Product/6
  Product/1 -> [Fx]
  Constant1/1 -> Product1/1
  [Cy] -> Product1/2
  [r_air] -> Product1/3
  [Vw] -> Product1/4
  [Vw] -> Product1/5
  [AL] -> Product1/6
  Product1/1 -> [Fy]
  Constant3/1 -> Product3/1
  [Cxy] -> Product3/2
  [r_air] -> Product3/3
  [Vw] -> Product3/4
  [Vw] -> Product3/5
  [AL] -> Product3/6
  [LOA] -> Product3/7
  Product3/1 -> transform z-downwards/1
  Mux1/1 -> F_wind/1
  Cx/1 -> [Cx]
  density of air/1 -> [r_air]
  velocity of the wind/1 -> [Vw]
  "LOA: overall length "/1 -> [LOA]
  AL: lateral projected area/1 -> [AL]
  Cy/1 -> [Cy]
  Cxy/1 -> [Cxy]
  AT: transverse projected area1/1 -> [AT]
  [Fx] -> Mux1/1
  [Fy] -> Mux1/2
  Constant4/1 -> Mux1/3
  Constant5/1 -> Mux1/4
  Constant6/1 -> Mux1/5
  [Mz] -> Mux1/6
  transform z-downwards/1 -> [Mz]

== system Chapter_4_Section_3_Model/Ship_Model/Ship Dynamics with Environmental Forces and Memory Effect/Buoyancy_Forces/Subsystem/wave elevation from multiple frequencies/Seakeeping motion of the ship from RAO's and wave spectrum  ==
  note: Note: the nb of itterations in the while loop corresponds to the nb of frequencies considered
  IC : Inport
  X : Inport  Port=2
  Y : Inport  Port=3
  t : Inport  Port=4
  ksi : Inport  Port=5
  Constant1 : Constant  Value=k_wave
  Constant2 : Constant  Value=S_wave
  Constant3 : Constant  Value=phase
  Constant4 : Constant  Value=w_star
  Embedded MATLAB Function : MATLAB Function  TreatAsAtomicUnit=on
  Embedded MATLAB Function1 : MATLAB Function  TreatAsAtomicUnit=on
  Embedded MATLAB Function2 : MATLAB Function  TreatAsAtomicUnit=on
  Embedded MATLAB Function3 : MATLAB Function  TreatAsAtomicUnit=on
  Memory1 : Memory  InheritSampleTime=on
  Read Me : simulink/Model-Wide Utilities/DocBlock  DocumentType=Text
  "Sea wave elevation from " : Subsystem
  Sum1 : Sum  Inputs=|+|+|
  While Iterator : WhileIterator  MaxIters=20  WhileBlockType=do-while  ResetStates=reset  ShowIterationPort=on  OutputDataType=double
  taw : Outport
  wires:
  While Iterator/1 -> [index]
  IC/1 -> While Iterator/1
  [index] -> Embedded MATLAB Function/1(index)
  Constant4/1 -> Embedded MATLAB Function/2(A)
  Embedded MATLAB Function/1(y) -> [w_star_i]
  [index] -> Embedded MATLAB Function1/1(index)
  Constant3/1 -> Embedded MATLAB Function1/2(A)
  Embedded MATLAB Function1/1(y) -> [phase_i]
  [index] -> Embedded MATLAB Function2/1(index)
  Constant1/1 -> Embedded MATLAB Function2/2(A)
  Embedded MATLAB Function2/1(y) -> [k_wave_i]
  [w_star_i] -> "Sea wave elevation from "/1(w_star)
  [k_wave_i] -> "Sea wave elevation from "/2(k_wave)
  [phase_i] -> "Sea wave elevation from "/3(phase)
  X/1 -> "Sea wave elevation from "/4(X)
  Y/1 -> "Sea wave elevation from "/5(Y)
  "Sea wave elevation from "/1(Sea wave Elevation(m)) -> Sum1/1
  Sum1/1 -> taw/1, Memory1/1
  Memory1/1 -> Sum1/2
  t/1 -> "Sea wave elevation from "/6(t)
  [S_i] -> "Sea wave elevation from "/7(S_power of ith wave)
  [index] -> Embedded MATLAB Function3/1(index)
  Constant2/1 -> Embedded MATLAB Function3/2(A)
  Embedded MATLAB Function3/1(y) -> [S_i]
  ksi/1 -> "Sea wave elevation from "/8(ksi)

== system Chapter_4_Section_3_Model/Ship_Model/Ship Dynamics with Environmental Forces and Memory Effect/Buoyancy_Forces/Subsystem/wave elevation from multiple frequencies1/Seakeeping motion of the ship from RAO's and wave spectrum  ==
  note: Note: the nb of itterations in the while loop corresponds to the nb of frequencies considered
  IC : Inport
  X : Inport  Port=2
  Y : Inport  Port=3
  t : Inport  Port=4
  ksi : Inport  Port=5
  Constant1 : Constant  Value=k_wave
  Constant2 : Constant  Value=S_wave
  Constant3 : Constant  Value=phase
  Constant4 : Constant  Value=w_star
  Embedded MATLAB Function : MATLAB Function  TreatAsAtomicUnit=on
  Embedded MATLAB Function1 : MATLAB Function  TreatAsAtomicUnit=on
  Embedded MATLAB Function2 : MATLAB Function  TreatAsAtomicUnit=on
  Embedded MATLAB Function3 : MATLAB Function  TreatAsAtomicUnit=on
  Memory1 : Memory  InheritSampleTime=on
  Read Me : simulink/Model-Wide Utilities/DocBlock  DocumentType=Text
  "Sea wave elevation from " : Subsystem
  Sum1 : Sum  Inputs=|+|+|
  While Iterator : WhileIterator  MaxIters=20  WhileBlockType=do-while  ResetStates=reset  ShowIterationPort=on  OutputDataType=double
  taw : Outport
  wires:
  While Iterator/1 -> [index]
  IC/1 -> While Iterator/1
  [index] -> Embedded MATLAB Function/1(index)
  Constant4/1 -> Embedded MATLAB Function/2(A)
  Embedded MATLAB Function/1(y) -> [w_star_i]
  [index] -> Embedded MATLAB Function1/1(index)
  Constant3/1 -> Embedded MATLAB Function1/2(A)
  Embedded MATLAB Function1/1(y) -> [phase_i]
  [index] -> Embedded MATLAB Function2/1(index)
  Constant1/1 -> Embedded MATLAB Function2/2(A)
  Embedded MATLAB Function2/1(y) -> [k_wave_i]
  [w_star_i] -> "Sea wave elevation from "/1(w_star)
  [k_wave_i] -> "Sea wave elevation from "/2(k_wave)
  [phase_i] -> "Sea wave elevation from "/3(phase)
  X/1 -> "Sea wave elevation from "/4(X)
  Y/1 -> "Sea wave elevation from "/5(Y)
  "Sea wave elevation from "/1(Sea wave Elevation(m)) -> Sum1/1
  Sum1/1 -> taw/1, Memory1/1
  Memory1/1 -> Sum1/2
  t/1 -> "Sea wave elevation from "/6(t)
  [S_i] -> "Sea wave elevation from "/7(S_power of ith wave)
  [index] -> Embedded MATLAB Function3/1(index)
  Constant2/1 -> Embedded MATLAB Function3/2(A)
  Embedded MATLAB Function3/1(y) -> [S_i]
  ksi/1 -> "Sea wave elevation from "/8(ksi)
